simulink model "pendulumSim"  (R2026a)
settings: Solver=FixedStepAuto  StopTime=10
values from neighbouring files (symbols this model uses):
  b = 2*(m*g*J*L)^0.5    (= 6.32455532034)    [pendulumScript.m]
  g = 10    [pendulumScript.m]
  J = m*L^2    (= 1)    [pendulumScript.m]
  L = 1    [pendulumScript.m]
  m = 2    [Spring.m]    (also in SystemModelling.m = 3; pendulumScript.m = 1)
settings Model: Creator=Lenovo LOQ  LastModifiedBy=Lenovo LOQ

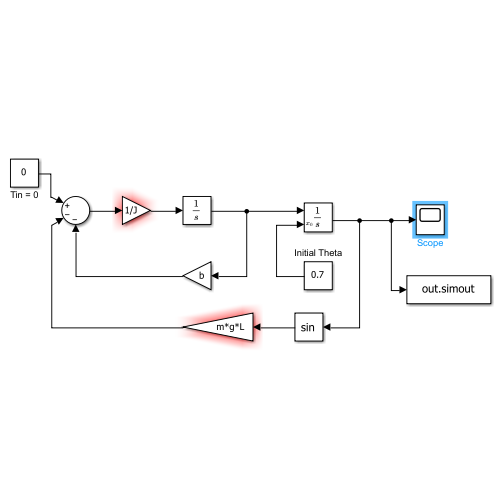
[thumbnail: Simulink's stored preview of the top-level diagram]
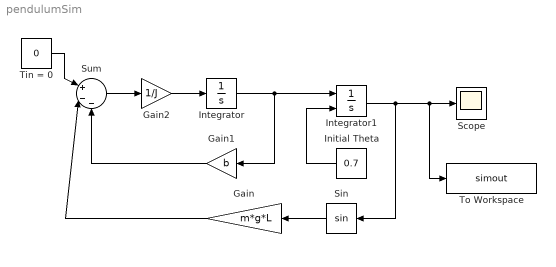
== system pendulumSim ==
  Gain : Gain  Gain=m*g*L
  Gain1 : Gain  Gain=b
  Gain2 : Gain  Gain=1/J
  Initial Theta : Constant  Value=0.7
  Integrator : Integrator
  Integrator1 : Integrator  InitialConditionSource=external
  Scope : Scope
      settings: ActiveDisplayYMinimum=-6.13955333457602E+31  ActiveDisplayYMaximum=2.3739371660385582E+31
  Sin : Trigonometry
  Sum : Sum  Inputs=|+--
  Tin = 0 : Constant  Value=0
  To Workspace : ToWorkspace  VariableName=simout  SaveFormat=Timeseries  SampleTime=-1
  wires:
  Initial Theta/1 -> Integrator1/2
  Integrator/1 -> Gain1/1, Integrator1/1
  Integrator1/1 -> To Workspace/1, Scope/1, Sin/1
  Sin/1 -> Gain/1
  Gain/1 -> Sum/2
  Tin = 0/1 -> Sum/1
  Gain1/1 -> Sum/3
  Gain2/1 -> Integrator/1
  Sum/1 -> Gain2/1
